simulink library "lib_PoseErrorCalulator"  (R2017b)
settings: Solver=VariableStepAuto  StartTime=0.0  StopTime=10.0  RelTol=1e-3
settings Model: Creator=muralikarnam  LastModifiedBy=muralikarnam

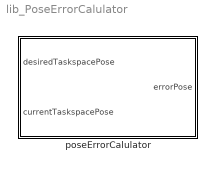
== system lib_PoseErrorCalulator ==
  poseErrorCalulator : MATLAB Function  TreatAsAtomicUnit=on

== matlab function lib_PoseErrorCalulator/poseErrorCalulator ==
  data: desiredTaskspacePose input double size=[4 4]; errorPose output double size=[6 1]; currentTaskspacePose input double size=[4 4]
%#codegen
function errorPose = poseErrorCalulator(desiredTaskspacePose, currentTaskspacePose)

errorPose = fun_PoseErrorCalulator(desiredTaskspacePose, currentTaskspacePose);

end
